simulink model "modelado_ANFIS"  (R2024b)
settings: Solver=VariableStepAuto  StartTime=0.0  StopTime=20  RelTol=1e-3
settings Model: Creator=user  LastModifiedBy=user

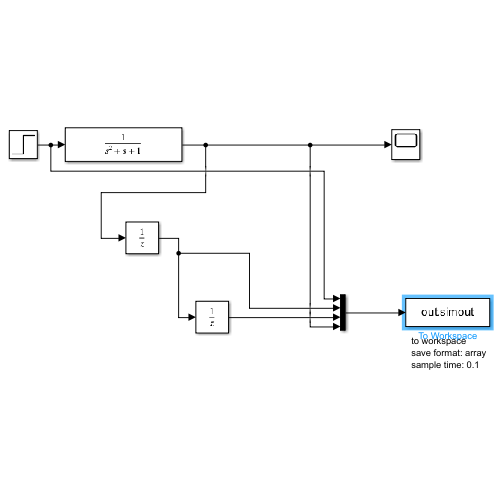
[thumbnail: Simulink's stored preview of the top-level diagram]
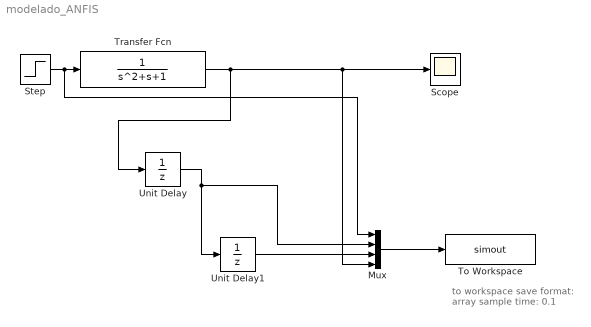
== system modelado_ANFIS ==
  note: to workspace
      | save format: array
      | sample time: 0.1
  Mux : Mux
  Scope : Scope
  Step : Step  SampleTime=0
  To Workspace : ToWorkspace  VariableName=simout  SampleTime=0.1
  Transfer Fcn : TransferFcn  Denominator=[1 1 1]
  Unit Delay : UnitDelay  SampleTime=-1  HasFrameUpgradeWarning=on
  Unit Delay1 : UnitDelay  SampleTime=-1  HasFrameUpgradeWarning=on
  wires:
  Transfer Fcn/1 -> Unit Delay/1, Mux/4, Scope/1
  Unit Delay/1 -> Unit Delay1/1, Mux/2
  Unit Delay1/1 -> Mux/3
  Step/1 -> Mux/1, Transfer Fcn/1
  Mux/1 -> To Workspace/1
